simulink subsystem "Puls"  (R2019b)
settings: Solver=VariableStepAuto  StartTime=0.0  StopTime=10.0  RelTol=1e-3
InitFcn:
  | %% DSPBuilder Start
  | alt_dspbuilder_update_model(bdroot)
  | %% DSPBuilder End
StartFcn:
  | %% DSPBuilder Start
  | alt_dspbuilder_hdlimport_prepare_for_simulation(bdroot)
  | %% DSPBuilder End
libraries: allblocks_alteradspbuilder2 x3
settings Model: Creator=vboxuser  LastModifiedBy=vboxuser

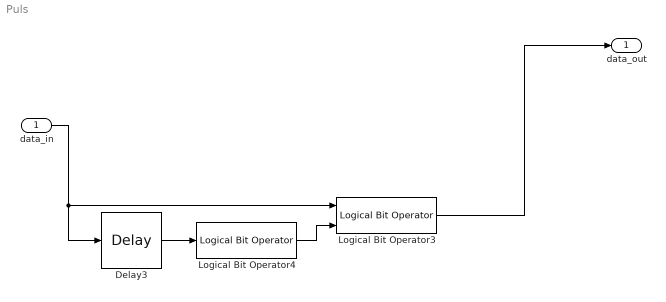
== system Puls ==
  data_in : Inport
  Delay3 : allblocks_alteradspbuilder2/Delay  pipeline=1  pipeline_display=1  ClockPhase=1  use_ena=off  use_sclr=off  allowFloatingPointOverride=on  logOutputs=off  logFile=C:\Users\vboxuser\Documents\MATLAB\serializer\system2\tb_matcher_simu_old\matcher%5Fsimu%5Fold_Subsystem_Subsystem_Delay3.fixedpointlog  use_init=off  reset_value=1
  Logical Bit Operator3 : allblocks_alteradspbuilder2/Logical Bit Operator  LogicalOperator=AND  user_inputs=2  pipeline_display=0
  Logical Bit Operator4 : allblocks_alteradspbuilder2/Logical Bit Operator  LogicalOperator=NOT  user_inputs=2  pipeline_display=0
  data_out : Outport
  wires:
  Logical Bit Operator4/1 -> Logical Bit Operator3/2
  Delay3/1 -> Logical Bit Operator4/1
  data_in/1 -> Logical Bit Operator3/1, Delay3/1
  Logical Bit Operator3/1 -> data_out/1
